simulink model "bulrpid"  (R2023a)
settings: Solver=VariableStepAuto  StartTime=0.0  StopTime=20  RelTol=1e-3
libraries: fuzblock x1
settings Model: Creator=belov  LastModifiedBy=belov
settings SolverCC: MaxConsecutiveMinStep=1000000

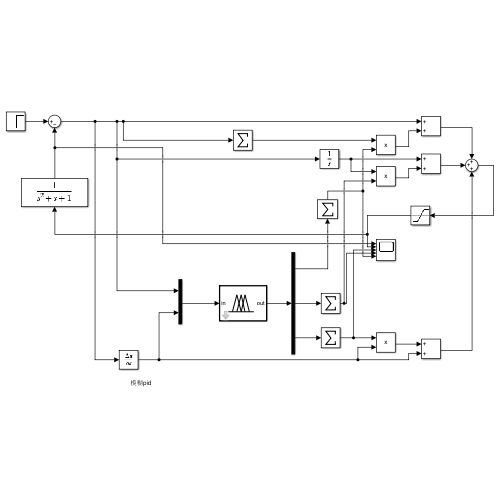
[thumbnail: Simulink's stored preview of the top-level diagram]
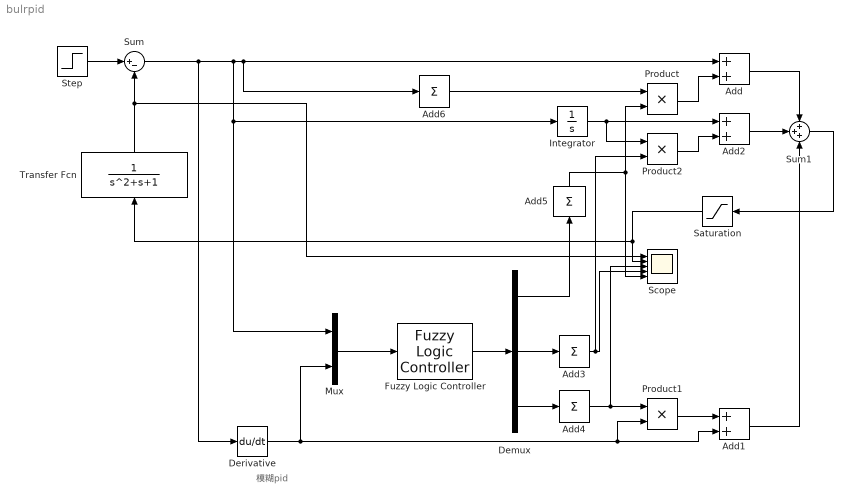
== system bulrpid ==
  note: 模糊pid
  Add : Sum
  Add1 : Sum
  Add2 : Sum
  Add{3..6} (4 alike) : Sum  Inputs=+
  Demux : Demux  Outputs=3
  Derivative : Derivative
  Fuzzy Logic Controller : fuzblock/Fuzzy Logic  Controller  FIS='pidbulr.fis'  OutputSampleNumber=101  DataType=double  FuzzifiedInputs=off  RuleFiringStrengths=off  RuleOutputs=off  AggregatedOutputs=off  SimulateUsing=Code generation  OutOfRangeInputValueMessage=warning  NoRuleFiredMessage=warning  EmptyOutputFuzzySetMessage=warning
  Integrator : Integrator
  Mux : Mux  Inputs=2
  Product : Product
  Product1 : Product
  Product2 : Product
  Saturation : Saturate  UpperLimit=5  LowerLimit=-5
  Scope : Scope  NumInputPorts=5
  Step : Step  SampleTime=0
  Sum : Sum  Inputs=|+-
  Sum1 : Sum  Inputs=+++
  Transfer Fcn : TransferFcn  Denominator=[1 1 1]
  wires:
  Step/1 -> Sum/1
  Fuzzy Logic Controller/1 -> Demux/1
  Sum1/1 -> Saturation/1
  Sum/1 -> Integrator/1, Mux/1, Add/1, Add6/1, Derivative/1
  Transfer Fcn/1 -> Sum/2, Scope/1
  Mux/1 -> Fuzzy Logic Controller/1
  Derivative/1 -> Product1/2, Add1/2, Mux/2
  Add6/1 -> Product/1
  Add4/1 -> Product1/1, Scope/3
  Demux/1 -> Add5/1
  Demux/2 -> Add3/1
  Demux/3 -> Add4/1
  Integrator/1 -> Add2/1, Product2/1
  Add5/1 -> Scope/5, Product/2
  Add3/1 -> Product2/2, Scope/4
  Product/1 -> Add/2
  Product2/1 -> Add2/2
  Product1/1 -> Add1/1
  Saturation/1 -> Scope/2, Transfer Fcn/1
  Add/1 -> Sum1/1
  Add2/1 -> Sum1/2
  Add1/1 -> Sum1/3
